simulink model "Vehicle1DBasic_testHarness"  (R2020a)
settings: Solver=VariableStepAuto  StartTime=0.0  StopTime=120  RelTol=1e-3  AbsTol=1e-3
PreLoadFcn:
  | Vehicle1DBasic_testParams
libraries: fl_lib x5, nesl_utility x2
settings Model: EnablePacing=on  Creator=isaacito  LastModifiedBy=isaacito
settings SolverCC: AutoScaleAbsTol=off
settings SimscapeCC: SimscapeLogType=local  SimscapeLogSimulationStatistics=on  SimscapeLogToSDI=on  SimscapeLogLimitData=off

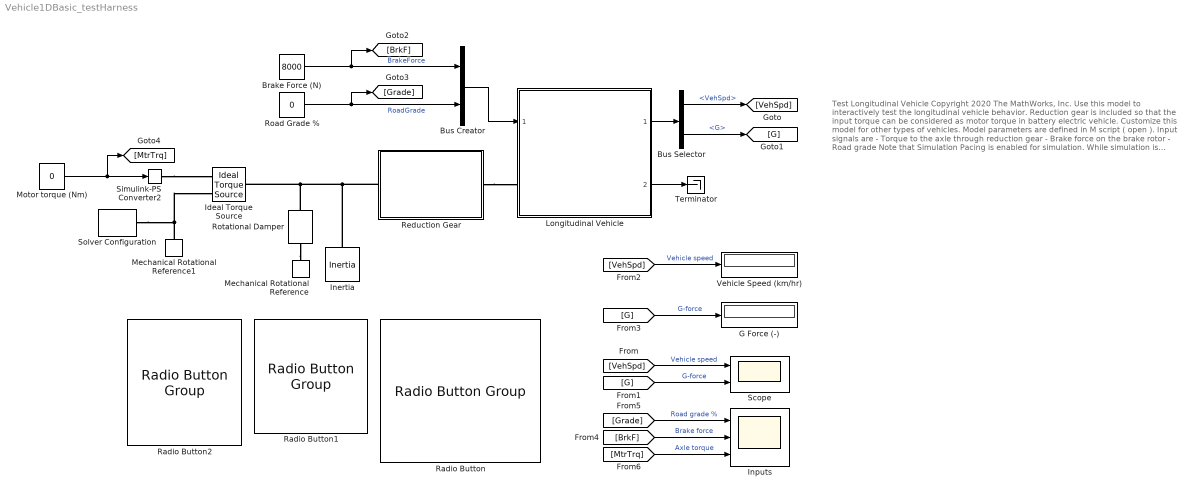
== system Vehicle1DBasic_testHarness ==
  note: Test Longitudinal Vehicle
      |
      | Copyright 2020 The MathWorks, Inc.
      |
      | Use this model to interactively test the longitudinal vehicle
      | behavior. Reduction gear is included so that the input torque
      | can be considered as motor torque in battery electric vehicle.
      | Customize this model for other types of vehicles.
      |
      | Model parameters are defined in M script ( open ).
      |
      | Input signals are
      |
      | - Torque to the axle through reduction gear
      | - Brake force on the brake rotor
      | - Road grade
      |
      | Note that Simulation Pacing is enabled for simulation. While
      | simulation is running, select torque, brake force, and road
      | grade in radio button, and observe the vehicle speed.
      | Input and output signal are also logged during simulation.
      | Use Data Inspector to plot the logged signals.
  Brake Force (N) : Constant  Value=8000
  Bus Creator : BusCreator  Inputs=2
  Bus Selector : BusSelector  OutputSignals=VehSpd,G
  G Force (-) : Display
  Ideal Torque Source : fl_lib/Mechanical/Mechanical Sources/Ideal Torque Source
  Inertia : fl_lib/Mechanical/Rotational Elements/Inertia  inertia=0.01 kg*m^2  w_specify=off  w_priority=High  w=0 rad/s  w_nominal_specify=off  w_nominal_unit=rad/s  w_nominal_value=1  t_specify=off  t_priority=None  t=0 N*m  t_nominal_specify=off  t_nominal_unit=N*m  t_nominal_value=1
      settings: AttributesFormatString=%<inertia> %<inertia_unit>
  Inputs : Scope  NumInputPorts=3
  Longitudinal Vehicle : Subsystem  ReferencedSubsystem=Vehicle1DBasicRefSub
  Mechanical Rotational Reference : fl_lib/Mechanical/Rotational Elements/Mechanical Rotational Reference
  Mechanical Rotational Reference1 : fl_lib/Mechanical/Rotational Elements/Mechanical Rotational Reference
  Motor torque (Nm) : Constant  Value=0
  Radio Button : RadioButtonGroup  SelectedLabel=0  ButtonGroupName=Group
      settings: Values={{'0', 'Grade 5 = 2.9 deg uphill', 'Grade 10 = 5.7 deg uphill', 'Grade 30 = 16.7 deg uphill', 'Grade -5 = -2.9 deg downhill', 'Grade -10 = -5.7 deg downhill', 'Grade -30 = -16.7 deg downhill'}, [0 5 10 30 -5 -10 -30]}
  Radio Button1 : RadioButtonGroup  SelectedLabel=8000 N  ButtonGroupName=Group
      settings: Values={{'0', '1000 N', '2000 N', '4000 N', '8000 N'}, [0 1000 2000 4000 8000]}
  Radio Button2 : RadioButtonGroup  SelectedLabel=0  ButtonGroupName=Group
      settings: Values={{'0', '100 N*m', '200 N*m', '400 N*m', '-100 N*m', '-200 N*m'}, [0 100 200 400 -100 -200]}
  Reduction Gear : Subsystem  ReferencedSubsystem=ReducerBasicRefSub
  Road Grade % : Constant  Value=0
  Rotational Damper : fl_lib/Mechanical/Rotational Elements/Rotational Damper  D=0.001 N*m/(rad/s)  w_specify=off  w_priority=None  w=0 rad/s  w_nominal_specify=off  w_nominal_unit=rad/s  w_nominal_value=1  t_specify=off  t_priority=None  t=0 N*m  t_nominal_specify=off  t_nominal_unit=N*m  t_nominal_value=1
      settings: AttributesFormatString=%<D> %<D_unit>
  Scope : Scope  NumInputPorts=2
  Simulink-PS Converter2 : nesl_utility/Simulink-PS Converter  PhysicalDomain=network_engine_domain  SubClassName=ps_input  LeftPortType=input  RightPortType=output  PseudoPeriodic=off  Frequencies=[]  NoiseDistribution=none  NoiseParameters=[]  Unit=N*m  AffineConversion=off  FilteringAndDerivatives=provide  SimscapeFilterOrder=1  InputFilterTimeConstant=0.001  UdotUserProvided=0
  Solver Configuration : nesl_utility/Solver Configuration  PhysicalDomain=network_engine_domain  SubClassName=solver  LeftPortType=input  RightPortType=generic  Tones=[]  Harmonics=[]  SimulateNoise=off  Profile=off  UseLocalSampling=off  EnableSwitchedLinearOptims=on  FrequencyDomain=off  UseCCode=off  RelTol=0.001  AbsTol=1e-06  MinStep=1e-09  ToWorkspace=off  RevertToSquareIcSolve=off  NumHomotopyIterations=100  PhasorMode=off  PhasorModeNumHarmonics=1  DoDC=off  ResidualTolerance=1e-09  UseLocalSolver=off  LocalSolverChoice=NE_BACKWARD_EULER_ADVANCER  LocalSolverSampleTime=0.001  DoFixedCost=off  MaxNonlinIter=3  MaxModeIter=2  LinearAlgebra=auto  EquationFormulation=NE_TIME_EF  DelaysMemoryBudget=1024  AutomaticFiltering=on  FilteringTimeConstant=0.001  PartitionStorageMethod=AS_NEEDED  PartitionMemoryBudget=1024  PartitionMethod=ROBUST
      settings: AttributesFormatString=Local solver %<UseLocalSolver>
  Terminator : Terminator
  Vehicle Speed (km/hr) : Display
  wires:
  Motor torque (Nm)/1 -> [MtrTrq], Simulink-PS Converter2/1
  [G] -> Scope/2  "G-force"
  [VehSpd] -> Scope/1  "Vehicle speed"
  Bus Selector/1 -> [VehSpd]  "<VehSpd>"
  Bus Selector/2 -> [G]  "<G>"
  [VehSpd] -> Vehicle Speed (km/hr)/1  "Vehicle speed"
  [G] -> G Force (-)/1  "G-force"
  Brake Force (N)/1 -> [BrkF], Bus Creator/1  "BrakeForce"
  Road Grade %/1 -> [Grade], Bus Creator/2  "RoadGrade"
  [Grade] -> Inputs/1  "Road grade %"
  [BrkF] -> Inputs/2  "Brake force"
  [MtrTrq] -> Inputs/3  "Axle torque"
  Longitudinal Vehicle/2 -> Terminator/1
  Longitudinal Vehicle/1 -> Bus Selector/1
  Bus Creator/1 -> Longitudinal Vehicle/1
  connections:
  Inertia/LConn1 -- Reduction Gear/LConn1 -- Rotational Damper/LConn1 -- Ideal Torque Source/LConn1
  Rotational Damper/RConn1 -- Mechanical Rotational Reference/LConn1
  Simulink-PS Converter2/RConn1 -- Ideal Torque Source/RConn1
  Mechanical Rotational Reference1/LConn1 -- Solver Configuration/RConn1 -- Ideal Torque Source/RConn2
  Reduction Gear/RConn1 -- Longitudinal Vehicle/LConn1
